simulink model "pend"  (R2021b)
settings: Solver=VariableStepAuto  StartTime=0.0  StopTime=100.0  MaxStep=0.01  RelTol=1e-3
undefined symbols (not defined in the file): b, g, J, l, m
libraries: simulink_extras x1
settings Model: Creator=vladimirberman  LastModifiedBy=vladimirberman

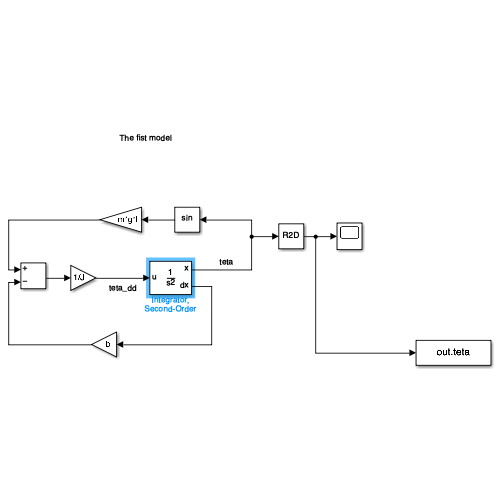
[thumbnail: Simulink's stored preview of the top-level diagram]
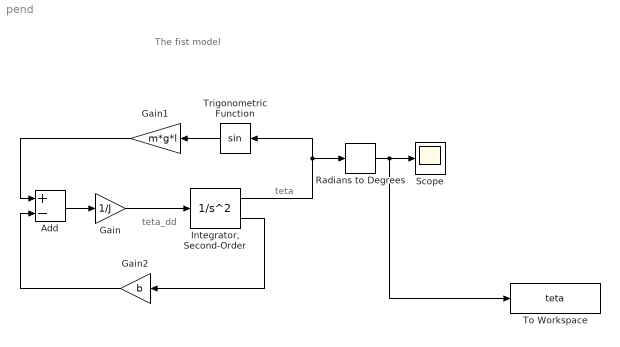
== system pend ==
  note: teta
  note: teta_dd
  note: The fist model
  Add : Sum  Inputs=+-
  Gain : Gain  Gain=1/J
  Gain1 : Gain  Gain=m*g*l
  Gain2 : Gain  Gain=b
  "Integrator, Second-Order" : SecondOrderIntegrator  ICX=0.01
  Radians to Degrees : simulink_extras/Transformations/Radians to Degrees
  Scope : Scope
  To Workspace : ToWorkspace  VariableName=teta  SampleTime=-1
  Trigonometric Function : Trigonometry
  wires:
  Gain/1 -> "Integrator, Second-Order"/1
  "Integrator, Second-Order"/1 -> Trigonometric Function/1, Radians to Degrees/1
  Trigonometric Function/1 -> Gain1/1
  Add/1 -> Gain/1
  Gain1/1 -> Add/1
  Gain2/1 -> Add/2
  "Integrator, Second-Order"/2 -> Gain2/1
  Radians to Degrees/1 -> To Workspace/1, Scope/1
